simulink model "IEEE_9bus_new_o"  (R2024a)
settings: Solver=ode45  StartTime=0.0  StopTime=60/60  RelTol=1e-3  EnableMultiTasking=on
PreLoadFcn:
  | faultType = "ABCG";
  | faultLineStr = "Line 7-8";
  | faultDistance = 50;
  | L78_Length = 50;
  | L89_Length = 50;
  | L96_Length = 50;
  | L64_Length = 50;
  | L45_Length = 50;
  | L57_Length = 50;
  | 
  | mdl = load('lineIdentificationModel.mat');
  | lineMdl = mdl.treeModel;
  | 
  | mdl = load('typeIdentificationModelV2.mat');
  | typeMdl = mdl.treeModel;
  | 
  | mdl = load('faultLocationModel.mat');
  | locationMdl = mdl.treeModel;
libraries: dspstat3 x36, simulink x24, spsThreePhasePISectionLineLib x12, spsThreePhaseVIMeasurementLib x12, spsLoadFlowBusLib x9, spsThreePhaseFaultLib x6, jailib x3, spsThreePhaseSourceLib x3, spsThreePhaseTransformerTwoWindingsLib x3, statsLibrary x3, spsThreePhaseBreakerLib x3, sps_lib x1
(part 1 of 3)
settings Model: Creator=jp536285  LastModifiedBy=USER
settings SolverCC: AlgebraicLoopSolver=TrustRegion
settings DataIOCC: LimitDataPoints=on  SaveFormat=Array  ReturnWorkspaceOutputs=off
settings OptimizationCC: LifeSpan=inf
settings DebuggingCC: UnderspecifiedInitializationDetection=Classic  MergeDetectMultiDrivingBlocksExec=none  SolverPrmCheckMsg=warning  StateNameClashWarn=warning  SFUnexpectedBacktrackingDiag=warning  SFNoUnconditionalDefaultTransitionDiag=warning  SFExecutionAtInitializationDiag=none  ArithmeticOperatorsInVariantConditions=warning
settings HardwareCC: ProdBitPerPointer=32  ProdBitPerSizeT=32  ProdBitPerPtrDiffT=32  ProdLargestAtomicFloat=None  ProdIntDivRoundTo=Undefined  ProdEndianess=Unspecified  ProdWordSize=32  ProdHWDeviceType=32-bit Generic
settings ModelReferenceCC: EnableParallelModelReferenceBuilds=on  ParallelModelReferenceMATLABWorkerInit=Copy Base Workspace
settings SFSimCC: SimUseLocalCustomCode=off  CustomCodeUndefinedFunction=UseInterfaceOnly
settings RTWCC: RTWUseLocalCustomCode=off  GPUComputeCapability=3.5
settings CodeAppCC: StateflowObjectComments=on
settings GRTTargetCC: TargetLangStandard=C89/C90 (ANSI)
settings ConfigComp: CovMetricSettings=dw  CovSaveCumulativeToWorkspaceVar=on  CovSaveSingleToWorkspaceVar=on  CovExternalEMLEnable=off
settings SimscapeCC: SimscapeNormalizeSystem=off

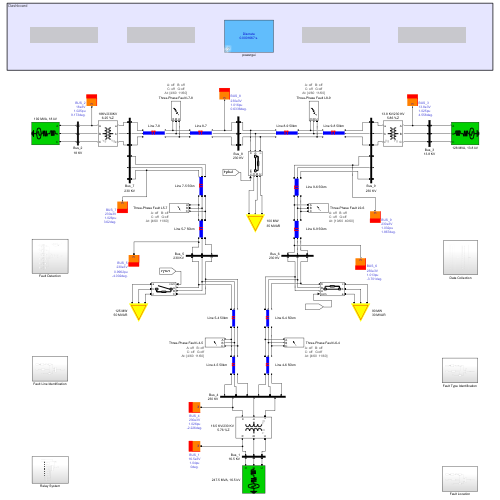
[thumbnail: Simulink's stored preview of the top-level diagram]
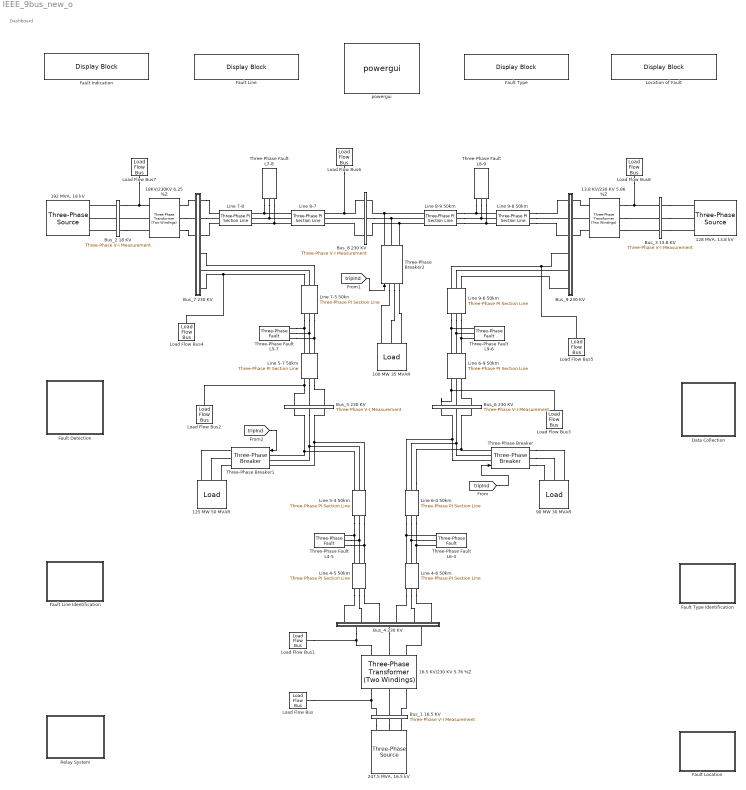
== system IEEE_9bus_new_o ==
  note: Dashboard
  " Line 4-6 50km" : spsThreePhasePISectionLineLib/Three-Phase PI Section Line  LConnTagsString=a|b|c  RConnTagsString=A|B|C  Length=100-L64_Length  Frequency=60  Resistances=[ 0.08993 0.224825]  Inductances="[ 1.29e-3  3.22e-3]"  Capacitances=[7.922e-9 4.74e-9]  mask(Three-Phase PI Section Line){}
      mask Display:
      | % This is a new mask on top of the base mask.
      | % Use "View base mask" link below to see the base mask.
      | patch([0.0 0.0 1 1 0.0 0.0 ],[0.4 0.7 0.7 0.4 0.4 0.7],[0 0 1]);
      | patch([0.4 0.4 0.42 0.42],[0.4 0.75 0.75 0.4],[1 0 0]);
      | patch([0.38 0.38 0.57 0.57],[0.7 0.75 0.75 0.7],[1 0 0]);
      | patch([0.53 0.53 0.55 0.55],[0.4 0.75 0.75 0.4],[1 0 0]);
  " Line 6-4 50km" : spsThreePhasePISectionLineLib/Three-Phase PI Section Line  LConnTagsString=a|b|c  RConnTagsString=A|B|C  Length=L64_Length  Frequency=60  Resistances=[ 0.08993 0.224825]  Inductances="[ 1.29e-3  3.22e-3]"  Capacitances=[7.922e-9 4.74e-9]  mask(Three-Phase PI Section Line){}
      mask Display:
      | % This is a new mask on top of the base mask.
      | % Use "View base mask" link below to see the base mask.
      | patch([0.0 0.0 1 1 0.0 0.0 ],[0.4 0.7 0.7 0.4 0.4 0.7],[0 0 1]);
      | patch([0.4 0.4 0.42 0.42],[0.4 0.75 0.75 0.4],[1 0 0]);
      | patch([0.38 0.38 0.57 0.57],[0.7 0.75 0.75 0.7],[1 0 0]);
      | patch([0.53 0.53 0.55 0.55],[0.4 0.75 0.75 0.4],[1 0 0]);
  " Line 6-9 50km" : spsThreePhasePISectionLineLib/Three-Phase PI Section Line  LConnTagsString=a|b|c  RConnTagsString=A|B|C  Length=100-L96_Length  Frequency=60  Resistances=[ 0.20631 0.5157]  Inductances="[ 2.38e-3  6.09e-3]"  Capacitances=[17.95e-9 10.55e-9]  mask(Three-Phase PI Section Line){}
      mask Display:
      | % This is a new mask on top of the base mask.
      | % Use "View base mask" link below to see the base mask.
      | patch([0.0 0.0 1 1 0.0 0.0 ],[0.4 0.7 0.7 0.4 0.4 0.7],[0 0 1]);
      | patch([0.4 0.4 0.42 0.42],[0.4 0.75 0.75 0.4],[1 0 0]);
      | patch([0.38 0.38 0.57 0.57],[0.7 0.75 0.75 0.7],[1 0 0]);
      | patch([0.53 0.53 0.55 0.55],[0.4 0.75 0.75 0.4],[1 0 0]);
  " Line 9-6 50km" : spsThreePhasePISectionLineLib/Three-Phase PI Section Line  LConnTagsString=a|b|c  RConnTagsString=A|B|C  Length=L96_Length  Frequency=60  Resistances=[ 0.20631 0.5157]  Inductances="[ 2.38e-3  6.09e-3]"  Capacitances=[17.95e-9 10.55e-9]  mask(Three-Phase PI Section Line){}
      mask Display:
      | % This is a new mask on top of the base mask.
      | % Use "View base mask" link below to see the base mask.
      | patch([0.0 0.0 1 1 0.0 0.0 ],[0.4 0.7 0.7 0.4 0.4 0.7],[0 0 1]);
      | patch([0.4 0.4 0.42 0.42],[0.4 0.75 0.75 0.4],[1 0 0]);
      | patch([0.38 0.38 0.57 0.57],[0.7 0.75 0.75 0.7],[1 0 0]);
      | patch([0.53 0.53 0.55 0.55],[0.4 0.75 0.75 0.4],[1 0 0]);
  100 MW 35 MVAR : jailib/Load  SystemSampleTime=-1  VariantActivationTime=update diagram  AllowFlexibleInterface=on  Latency=0  AutoFrameSizeCalculation=off
      link override Three-Phase Parallel RLC Load: NominalVoltage=230000  ActivePower=100e6  InductivePower=35e6
      settings: SourceProductName=Power Library
  125 MW 50 MVAR : jailib/Load  SystemSampleTime=-1  VariantActivationTime=update diagram  AllowFlexibleInterface=on  Latency=0  AutoFrameSizeCalculation=off
      link override Three-Phase Parallel RLC Load: NominalVoltage=230000  ActivePower=125e6  InductivePower=50e6
      settings: SourceProductName=Power Library
  "128 MVA, 13.8 kV" : spsThreePhaseSourceLib/Three-Phase Source  InternalConnection=Yg  VoltagePhases=off  Voltage=13800  PhaseAngle=0  Voltage_phases=[25e3 25e3 25e3]/sqrt(3)  PhaseAngles_phases=[0 -120 +120]  Frequency=60  NonIdealSource=on  SpecifyImpedance=on  Resistance=0.529  Inductance=0.0140  ShortCircuitLevel=128e6  BaseVoltage=13.8e3  XRratio=100000  BusType=PV  Pref=85000000  Qref=0  Prefabc=[10e3, 10e3, 10e3]  Qrefabc=[0, 0, 0]  Qmin=-inf  Qmax=inf
  13.8 KV/230 KV 5.86 %Z : spsThreePhaseTransformerTwoWindingsLib/Three-Phase Transformer (Two Windings)  Winding1Connection=Yg  Winding2Connection=Yg  CoreType=Three single-phase transformers  SetSaturation=off  Hysteresis=off  DataFile='hysteresis'  SetInitialFlux=off  Measurements=None  UNITS=pu  NominalPower=[ 100e6 , 60 ]  Winding1=[ 13.8e3 , 1e-6 , 0 ]  Winding2=[ 230e3 , 1e-6, 0.0586 ]  Rm=500  Lm=500  L0=0.5  Saturation=[ 0,0 ; 0.0024,1.2 ; 1.0,1.52 ]  InitialFluxes=[ 0.8 , -0.8 , 0.7 ]  BreakLoop=off  DiscreteSolver=Trapezoidal iterative  DataType=off  TransfoNumber=1
  "16.5 KV/230 KV 5.76 %Z     " : spsThreePhaseTransformerTwoWindingsLib/Three-Phase Transformer (Two Windings)  Winding1Connection=Yg  Winding2Connection=Yg  CoreType=Three single-phase transformers  SetSaturation=off  Hysteresis=off  DataFile='hysteresis'  SetInitialFlux=off  Measurements=None  UNITS=pu  NominalPower=[ 100e6 , 60 ]  Winding1=[ 16.5e3 , 1e-6, 0 ]  Winding2=[ 230e3 ,1e-6, 0.0576 ]  Rm=500  Lm=500  L0=0.5  Saturation=[ 0,0 ; 0.0024,1.2 ; 1.0,1.52 ]  InitialFluxes=[ 0.8 , -0.8 , 0.7 ]  BreakLoop=off  DiscreteSolver=Trapezoidal iterative  DataType=off  TransfoNumber=1
  18KV/230KV 6.25 %Z : spsThreePhaseTransformerTwoWindingsLib/Three-Phase Transformer (Two Windings)  Winding1Connection=Yg  Winding2Connection=Yg  CoreType=Three single-phase transformers  SetSaturation=off  Hysteresis=off  DataFile='hysteresis'  SetInitialFlux=off  Measurements=None  UNITS=pu  NominalPower=[ 100e6 , 60 ]  Winding1=[ 18e3 , 1e-6 , 0]  Winding2=[ 230e3 , 1e-6, 0.0625 ]  Rm=500  Lm=500  L0=0.5  Saturation=[ 0,0 ; 0.0024,1.2 ; 1.0,1.52 ]  InitialFluxes=[ 0.8 , -0.8 , 0.7 ]  BreakLoop=off  DiscreteSolver=Trapezoidal iterative  DataType=off  TransfoNumber=1
  "192 MVA, 18 kV" : spsThreePhaseSourceLib/Three-Phase Source  InternalConnection=Yg  VoltagePhases=off  Voltage=18000  PhaseAngle=0  Voltage_phases=[25e3 25e3 25e3]/sqrt(3)  PhaseAngles_phases=[0 -120 +120]  Frequency=60  NonIdealSource=on  SpecifyImpedance=on  Resistance=0.529  Inductance=0.0140  ShortCircuitLevel=192e6  BaseVoltage=18e3  XRratio=100000  BusType=PV  Pref=163000000  Qref=0  Prefabc=[10e3, 10e3, 10e3]  Qrefabc=[0, 0, 0]  Qmin=-inf  Qmax=inf
  "247.5 MVA, 16.5 kV" : spsThreePhaseSourceLib/Three-Phase Source  InternalConnection=Yg  VoltagePhases=off  Voltage=16500  PhaseAngle=0  Voltage_phases=[25e3 25e3 25e3]/sqrt(3)  PhaseAngles_phases=[0 -120 +120]  Frequency=60  NonIdealSource=on  SpecifyImpedance=on  Resistance=0.529  Inductance=0.0140  ShortCircuitLevel=247.5e6  BaseVoltage=16.5e3  XRratio=100000  BusType=swing  Pref=0  Qref=0  Prefabc=[10e3, 10e3, 10e3]  Qrefabc=[0, 0, 0]  Qmin=-Inf  Qmax=Inf
  90 MW 30 MVAR : jailib/Load  SystemSampleTime=-1  VariantActivationTime=update diagram  AllowFlexibleInterface=on  Latency=0  AutoFrameSizeCalculation=off
      settings: SourceProductName=Power Library
  Bus_1 16.5 KV : spsThreePhaseVIMeasurementLib/Three-Phase V-I Measurement  VoltageMeasurement=phase-to-ground  SetLabelV=on  LabelV=Vabc_1  Vpu=on  VpuLL=off  CurrentMeasurement=yes  SetLabelI=on  LabelI=Iabc_1  Ipu=on  Pbase=100e6  Vbase=16.5e3  OutputType=Complex  PhasorSimulation=off  PSBequivalent=0
  Bus_2 18 KV : spsThreePhaseVIMeasurementLib/Three-Phase V-I Measurement  VoltageMeasurement=phase-to-ground  SetLabelV=on  LabelV=Vabc_2  Vpu=on  VpuLL=off  CurrentMeasurement=yes  SetLabelI=on  LabelI=Iabc_2  Ipu=on  Pbase=100e6  Vbase=18e3  OutputType=Complex  PhasorSimulation=off  PSBequivalent=0
  Bus_3 13.8 KV : spsThreePhaseVIMeasurementLib/Three-Phase V-I Measurement  VoltageMeasurement=phase-to-ground  SetLabelV=on  LabelV=Vabc_3  Vpu=on  VpuLL=off  CurrentMeasurement=yes  SetLabelI=on  LabelI=Iabc_3  Ipu=on  Pbase=100e6  Vbase=13.8e3  OutputType=Complex  PhasorSimulation=off  PSBequivalent=0
  Bus_4 230 KV : Subsystem
  Bus_5 230 KV : spsThreePhaseVIMeasurementLib/Three-Phase V-I Measurement  VoltageMeasurement=phase-to-ground  SetLabelV=on  LabelV=Vabc_5  Vpu=on  VpuLL=off  CurrentMeasurement=yes  SetLabelI=on  LabelI=Iabc_5  Ipu=on  Pbase=100e6  Vbase=230e3  OutputType=Complex  PhasorSimulation=off  PSBequivalent=0
  Bus_6 230 KV : spsThreePhaseVIMeasurementLib/Three-Phase V-I Measurement  VoltageMeasurement=phase-to-ground  SetLabelV=on  LabelV=Vabc_6  Vpu=on  VpuLL=off  CurrentMeasurement=yes  SetLabelI=on  LabelI=Iabc_6  Ipu=on  Pbase=100e6  Vbase=230e3  OutputType=Complex  PhasorSimulation=off  PSBequivalent=0
  Bus_7 230 KV : Subsystem
  Bus_8 230 KV : spsThreePhaseVIMeasurementLib/Three-Phase V-I Measurement  VoltageMeasurement=phase-to-ground  SetLabelV=on  LabelV=Vabc_8  Vpu=on  VpuLL=off  CurrentMeasurement=yes  SetLabelI=on  LabelI=Iabc_8  Ipu=on  Pbase=100e6  Vbase=230e3  OutputType=Complex  PhasorSimulation=off  PSBequivalent=0
  Bus_9 230 KV : Subsystem
  Data Collection : Subsystem
  Fault Detection : Subsystem
  Fault Indication : DisplayBlock  LabelPosition=Hide  Transparency=1  Layout=Fill available space
  Fault Line : DisplayBlock  LabelPosition=Hide  Transparency=1
  Fault Line Identification : Subsystem
  Fault Location : Subsystem
  Fault Type : DisplayBlock  LabelPosition=Hide  Transparency=1
  Fault Type Identification : Subsystem
  "Line 4-5 50km " : spsThreePhasePISectionLineLib/Three-Phase PI Section Line  LConnTagsString=a|b|c  RConnTagsString=A|B|C  Length=L45_Length  Frequency=60  Resistances=[ 0.0529 0.13225]  Inductances="[ 1.192e-3  2.38e-3]"  Capacitances=[8.82e-9 5.188e-9]  mask(Three-Phase PI Section Line){}
      mask Display:
      | % This is a new mask on top of the base mask.
      | % Use "View base mask" link below to see the base mask.
      | patch([0.0 0.0 1 1 0.0 0.0 ],[0.4 0.7 0.7 0.4 0.4 0.7],[0 0 1]);
      | patch([0.4 0.4 0.42 0.42],[0.4 0.75 0.75 0.4],[1 0 0]);
      | patch([0.38 0.38 0.57 0.57],[0.7 0.75 0.75 0.7],[1 0 0]);
      | patch([0.53 0.53 0.55 0.55],[0.4 0.75 0.75 0.4],[1 0 0]);
  Line 5-4 50km : spsThreePhasePISectionLineLib/Three-Phase PI Section Line  LConnTagsString=a|b|c  RConnTagsString=A|B|C  Length=100-L45_Length  Frequency=60  Resistances=[ 0.0529 0.13225]  Inductances="[ 1.192e-3  2.38e-3]"  Capacitances=[8.82e-9 5.188e-9]  mask(Three-Phase PI Section Line){}
      mask Display:
      | % This is a new mask on top of the base mask.
      | % Use "View base mask" link below to see the base mask.
      | patch([0.0 0.0 1 1 0.0 0.0 ],[0.4 0.7 0.7 0.4 0.4 0.7],[0 0 1]);
      | patch([0.4 0.4 0.42 0.42],[0.4 0.75 0.75 0.4],[1 0 0]);
      | patch([0.38 0.38 0.57 0.57],[0.7 0.75 0.75 0.7],[1 0 0]);
      | patch([0.53 0.53 0.55 0.55],[0.4 0.75 0.75 0.4],[1 0 0]);
  Line 5-7 50km : spsThreePhasePISectionLineLib/Three-Phase PI Section Line  LConnTagsString=a|b|c  RConnTagsString=A|B|C  Length=L57_Length  Frequency=60  Resistances=[ 0.16928 0.4232]  Inductances="[ 2.259e-3  5.64e-3]"  Capacitances=[15.34e-9 9.025e-9]  mask(Three-Phase PI Section Line){}
      mask Display:
      | % This is a new mask on top of the base mask.
      | % Use "View base mask" link below to see the base mask.
      | patch([0.0 0.0 1 1 0.0 0.0 ],[0.4 0.7 0.7 0.4 0.4 0.7],[0 0 1]);
      | patch([0.4 0.4 0.42 0.42],[0.4 0.75 0.75 0.4],[1 0 0]);
      | patch([0.38 0.38 0.57 0.57],[0.7 0.75 0.75 0.7],[1 0 0]);
      | patch([0.53 0.53 0.55 0.55],[0.4 0.75 0.75 0.4],[1 0 0]);
  Line 7-5 50kn : spsThreePhasePISectionLineLib/Three-Phase PI Section Line  LConnTagsString=a|b|c  RConnTagsString=A|B|C  Length=100-L57_Length  Frequency=60  Resistances=[ 0.16928 0.4232]  Inductances="[ 2.259e-3  5.64e-3]"  Capacitances=[15.34e-9 9.025e-9]  mask(Three-Phase PI Section Line){}
      mask Display:
      | % This is a new mask on top of the base mask.
      | % Use "View base mask" link below to see the base mask.
      | patch([0.0 0.0 1 1 0.0 0.0 ],[0.4 0.7 0.7 0.4 0.4 0.7],[0 0 1]);
      | patch([0.4 0.4 0.42 0.42],[0.4 0.75 0.75 0.4],[1 0 0]);
      | patch([0.38 0.38 0.57 0.57],[0.7 0.75 0.75 0.7],[1 0 0]);
      | patch([0.53 0.53 0.55 0.55],[0.4 0.75 0.75 0.4],[1 0 0]);
  Line 7-8 : spsThreePhasePISectionLineLib/Three-Phase PI Section Line  LConnTagsString=a|b|c  RConnTagsString=A|B|C  Length=L78_Length  Frequency=60  Resistances=[0.044965 0.11241]  Inductances="[ 1.01e-3  2.02e-3]"  Capacitances=[7.471e-9 4.394e-9]  mask(Three-Phase PI Section Line){}
      mask Display:
      | % This is a new mask on top of the base mask.
      | % Use "View base mask" link below to see the base mask.
      | patch([0.0 0.0 1 1 0.0 0.0 ],[0.4 0.7 0.7 0.4 0.4 0.7],[0 0 1]);
      | patch([0.4 0.4 0.42 0.42],[0.4 0.75 0.75 0.4],[1 0 0]);
      | patch([0.38 0.38 0.57 0.57],[0.7 0.75 0.75 0.7],[1 0 0]);
      | patch([0.53 0.53 0.55 0.55],[0.4 0.75 0.75 0.4],[1 0 0]);
  Line 8-7 : spsThreePhasePISectionLineLib/Three-Phase PI Section Line  LConnTagsString=a|b|c  RConnTagsString=A|B|C  Length=100 - L78_Length  Frequency=60  Resistances=[0.044965 0.11241]  Inductances="[ 1.01e-3  2.02e-3]"  Capacitances=[7.471e-9 4.394e-9]  mask(Three-Phase PI Section Line){}
      mask Display:
      | % This is a new mask on top of the base mask.
      | % Use "View base mask" link below to see the base mask.
      | patch([0.0 0.0 1 1 0.0 0.0 ],[0.4 0.7 0.7 0.4 0.4 0.7],[0 0 1]);
      | patch([0.4 0.4 0.42 0.42],[0.4 0.75 0.75 0.4],[1 0 0]);
      | patch([0.38 0.38 0.57 0.57],[0.7 0.75 0.75 0.7],[1 0 0]);
      | patch([0.53 0.53 0.55 0.55],[0.4 0.75 0.75 0.4],[1 0 0]);
  Line 8-9 50km : spsThreePhasePISectionLineLib/Three-Phase PI Section Line  LConnTagsString=a|b|c  RConnTagsString=A|B|C  Length=L89_Length  Frequency=60  Resistances=[ 0.062951 0.15737]  Inductances="[ 1.414e-3  3.53e-3]"  Capacitances=[10.47e-9 6.15e-9]  mask(Three-Phase PI Section Line){}
      mask Display:
      | % This is a new mask on top of the base mask.
      | % Use "View base mask" link below to see the base mask.
      | patch([0.0 0.0 1 1 0.0 0.0 ],[0.4 0.7 0.7 0.4 0.4 0.7],[0 0 1]);
      | patch([0.4 0.4 0.42 0.42],[0.4 0.75 0.75 0.4],[1 0 0]);
      | patch([0.38 0.38 0.57 0.57],[0.7 0.75 0.75 0.7],[1 0 0]);
      | patch([0.53 0.53 0.55 0.55],[0.4 0.75 0.75 0.4],[1 0 0]);
  Line 9-8 50km : spsThreePhasePISectionLineLib/Three-Phase PI Section Line  LConnTagsString=a|b|c  RConnTagsString=A|B|C  Length=100-L89_Length  Frequency=60  Resistances=[ 0.062951 0.15737]  Inductances="[ 1.414e-3  3.53e-3]"  Capacitances=[10.47e-9 6.15e-9]  mask(Three-Phase PI Section Line){}
      mask Display:
      | % This is a new mask on top of the base mask.
      | % Use "View base mask" link below to see the base mask.
      | patch([0.0 0.0 1 1 0.0 0.0 ],[0.4 0.7 0.7 0.4 0.4 0.7],[0 0 1]);
      | patch([0.4 0.4 0.42 0.42],[0.4 0.75 0.75 0.4],[1 0 0]);
      | patch([0.38 0.38 0.57 0.57],[0.7 0.75 0.75 0.7],[1 0 0]);
      | patch([0.53 0.53 0.55 0.55],[0.4 0.75 0.75 0.4],[1 0 0]);
  Load Flow Bus : spsLoadFlowBusLib/Load Flow Bus  LConnTagsString=a  Phases=single  Connectors=on one side  ID=BUS_1  Vbase=16.5e3  Vref=1.04  Vangle=0  VLF=1.04  VLFb=1  VLFc=1  angleLF=0  angleLFb=0  angleLFc=0
      settings: AttributesFormatString=%<ID>\n%<Vbase>V\n%<VLF>pu\n%<angleLF>deg.
  Load Flow Bus1 : spsLoadFlowBusLib/Load Flow Bus  LConnTagsString=a  Phases=single  Connectors=on one side  ID=BUS_4  Vbase=230e3  Vref=1  Vangle=0  VLF=1.026  VLFb=1  VLFc=1  angleLF=-2.226  angleLFb=0  angleLFc=0
      settings: AttributesFormatString=%<ID>\n%<Vbase>V\n%<VLF>pu\n%<angleLF>deg.
  Load Flow Bus2 : spsLoadFlowBusLib/Load Flow Bus  LConnTagsString=a  Phases=single  Connectors=on one side  ID=BUS_5  Vbase=230e3  Vref=1  Vangle=0  VLF=0.9962  VLFb=1  VLFc=1  angleLF=-4.002  angleLFb=0  angleLFc=0
      settings: AttributesFormatString=%<ID>\n%<Vbase>V\n%<VLF>pu\n%<angleLF>deg.
  Load Flow Bus3 : spsLoadFlowBusLib/Load Flow Bus  LConnTagsString=a  Phases=single  Connectors=on one side  ID=BUS_6  Vbase=230e3  Vref=1  Vangle=0  VLF=1.013  VLFb=1  VLFc=1  angleLF=-3.701  angleLFb=0  angleLFc=0
      settings: AttributesFormatString=%<ID>\n%<Vbase>V\n%<VLF>pu\n%<angleLF>deg.
  Load Flow Bus4 : spsLoadFlowBusLib/Load Flow Bus  LConnTagsString=a  Phases=single  Connectors=on one side  ID=BUS_7  Vbase=230e3  Vref=1  Vangle=0  VLF=1.026  VLFb=1  VLFc=1  angleLF=3.62  angleLFb=0  angleLFc=0
      settings: AttributesFormatString=%<ID>\n%<Vbase>V\n%<VLF>pu\n%<angleLF>deg.
  Load Flow Bus5 : spsLoadFlowBusLib/Load Flow Bus  LConnTagsString=a  Phases=single  Connectors=on one side  ID=BUS_9  Vbase=230e3  Vref=1  Vangle=0  VLF=1.032  VLFb=1  VLFc=1  angleLF=1.867  angleLFb=0  angleLFc=0
      settings: AttributesFormatString=%<ID>\n%<Vbase>V\n%<VLF>pu\n%<angleLF>deg.
  Load Flow Bus6 : spsLoadFlowBusLib/Load Flow Bus  LConnTagsString=a  Phases=single  Connectors=on one side  ID=BUS_8  Vbase=230e3  Vref=1  Vangle=0  VLF=1.016  VLFb=1  VLFc=1  angleLF=0.6336  angleLFb=0  angleLFc=0
      settings: AttributesFormatString=%<ID>\n%<Vbase>V\n%<VLF>pu\n%<angleLF>deg.
  Load Flow Bus7 : spsLoadFlowBusLib/Load Flow Bus  LConnTagsString=a  Phases=single  Connectors=on one side  ID=BUS_2  Vbase=18e3  Vref=1.025  Vangle=0  VLF=1.025  VLFb=1  VLFc=1  angleLF=9.173  angleLFb=0  angleLFc=0
      settings: AttributesFormatString=%<ID>\n%<Vbase>V\n%<VLF>pu\n%<angleLF>deg.
  Load Flow Bus8 : spsLoadFlowBusLib/Load Flow Bus  LConnTagsString=a  Phases=single  Connectors=on one side  ID=BUS_3  Vbase=13.8e3  Vref=1.025  Vangle=0  VLF=1.025  VLFb=1  VLFc=1  angleLF=4.558  angleLFb=0  angleLFc=0
      settings: AttributesFormatString=%<ID>\n%<Vbase>V\n%<VLF>pu\n%<angleLF>deg.
  Location of Fault : DisplayBlock  LabelPosition=Hide  Transparency=1
  Relay System : Subsystem
  Three-Phase Breaker : spsThreePhaseBreakerLib/Three-Phase Breaker  InitialState=closed  SwitchA=off  SwitchB=off  SwitchC=off  SwitchTimes="[1/60  5/60]"  External=on  BreakerResistance=0.01  SnubberResistance=1e6  SnubberCapacitance=inf  Measurements=None
  Three-Phase Breaker1 : spsThreePhaseBreakerLib/Three-Phase Breaker  InitialState=open  SwitchA=off  SwitchB=off  SwitchC=off  SwitchTimes="[0/60  14/60]"  External=on  BreakerResistance=0.01  SnubberResistance=1e6  SnubberCapacitance=inf  Measurements=None
  Three-Phase Breaker2 : spsThreePhaseBreakerLib/Three-Phase Breaker  InitialState=closed  SwitchA=off  SwitchB=off  SwitchC=off  SwitchTimes="[1/60  5/60]"  External=on  BreakerResistance=0.01  SnubberResistance=1e6  SnubberCapacitance=inf  Measurements=None
  Three-Phase Fault L4-5 : spsThreePhaseFaultLib/Three-Phase Fault  InitialStates=0  FaultA=off  FaultB=off  FaultC=off  GroundFault=off  SwitchTimes="[4/60  11/60]"  External=off  SwitchStatus=NaN  FaultResistance=0.001  GroundResistance=0.01  SnubberResistance=1e6  SnubberCapacitance=inf  Measurements=None
      settings: AttributesFormatString=|
      | A: %<FaultA>   B: %<FaultB>
      | C: %<FaultC>   G:%<GroundFault>
      | At: %<SwitchTimes>
  Three-Phase Fault L5-7 : spsThreePhaseFaultLib/Three-Phase Fault  InitialStates=0  FaultA=off  FaultB=off  FaultC=off  GroundFault=off  SwitchTimes="[4/60  11/60]"  External=off  SwitchStatus=NaN  FaultResistance=0.001  GroundResistance=0.01  SnubberResistance=1e6  SnubberCapacitance=inf  Measurements=None
      settings: AttributesFormatString=|
      | A: %<FaultA>   B: %<FaultB>
      | C: %<FaultC>   G:%<GroundFault>
      | At: %<SwitchTimes>
  Three-Phase Fault L6-4 : spsThreePhaseFaultLib/Three-Phase Fault  InitialStates=0  FaultA=off  FaultB=off  FaultC=off  GroundFault=off  SwitchTimes="[4/60  11/60]"  External=off  SwitchStatus=NaN  FaultResistance=0.001  GroundResistance=0.01  SnubberResistance=1e6  SnubberCapacitance=inf  Measurements=None
      settings: AttributesFormatString=|
      | A: %<FaultA>   B: %<FaultB>
      | C: %<FaultC>   G:%<GroundFault>
      | At: %<SwitchTimes>
  Three-Phase Fault L7-8 : spsThreePhaseFaultLib/Three-Phase Fault  InitialStates=0  FaultA=off  FaultB=off  FaultC=off  GroundFault=off  SwitchTimes="[4/60  11/60]"  External=off  SwitchStatus=NaN  FaultResistance=0.001  GroundResistance=0.01  SnubberResistance=1e6  SnubberCapacitance=inf  Measurements=None
      settings: AttributesFormatString=|
      | A: %<FaultA>   B: %<FaultB>
      | C: %<FaultC>   G:%<GroundFault>
      | At: %<SwitchTimes>
  Three-Phase Fault L8-9 : spsThreePhaseFaultLib/Three-Phase Fault  InitialStates=0  FaultA=off  FaultB=off  FaultC=off  GroundFault=off  SwitchTimes="[4/60  11/60]"  External=off  SwitchStatus=NaN  FaultResistance=0.001  GroundResistance=0.01  SnubberResistance=1e6  SnubberCapacitance=inf  Measurements=None
      settings: AttributesFormatString=|
      | A: %<FaultA>   B: %<FaultB>
      | C: %<FaultC>   G:%<GroundFault>
      | At: %<SwitchTimes>
  Three-Phase Fault L9-6 : spsThreePhaseFaultLib/Three-Phase Fault  InitialStates=0  FaultA=off  FaultB=off  FaultC=off  GroundFault=off  SwitchTimes="[10/60  40/60]"  External=off  SwitchStatus=NaN  FaultResistance=0.001  GroundResistance=0.01  SnubberResistance=1e6  SnubberCapacitance=inf  Measurements=None
      settings: AttributesFormatString=|
      | A: %<FaultA>   B: %<FaultB>
      | C: %<FaultC>   G:%<GroundFault>
      | At: %<SwitchTimes>
  powergui : sps_lib/powergui  Priority=1  SimulationMode=Discrete  SampleTime=(1/6)*10^(-3)  frequency=60  Iterations=50  frequencyindice=60  Pbase=10e7  ErrMax=1e-05  UnitsV=kV  UnitsW=MW  buscounter=0  FunctionMessages=off  echomessages=off  EnableUseOfTLC=off  CurrentSourceSwitches=off  DisableSnubberDevices=off  DisableRonSwitches=off  DisableVfSwitches=off  DisplayEquations=off  AutomaticDiscreteSolvers=off  SolverType=Tustin  Interpol=off  ExternalGateDelay=off  methode=off  Ts=0  x0status=blocks  SPID=off  SwTol=0  HookPort=off  NonlinearTolerance=1e-4  nMaxIteration=100  ContinueOnMaxIteration=off  RestoreLinks=warning  ResistiveCurrentMeasurement=off  Frange=[0:2:500]  Ylog=off  Xlog=on  ShowGrid=off  save=off  variable=ZData  structure=0  ZoomFFT=off  StartTime=0.0  cycles=1  DisplayStyle=1  fundamental=60  FreqAxis=off  MaxFrequency=1000  frequencyindicesteady=1  RmsSteady=1  display=off
  wires:
  [tripInd] -> Three-Phase Breaker/1
  [tripInd] -> Three-Phase Breaker2/1
  [tripInd] -> Three-Phase Breaker1/1
  connections:
  Bus_2 18 KV/LConn2 -- "192 MVA, 18 kV"/RConn2
  18KV/230KV 6.25 %Z/LConn2 -- Bus_2 18 KV/RConn2
  18KV/230KV 6.25 %Z/RConn2 -- Bus_7 230 KV/LConn2
  Bus_2 18 KV/RConn1 -- Load Flow Bus7/LConn1 -- 18KV/230KV 6.25 %Z/LConn1
  Bus_2 18 KV/RConn3 -- 18KV/230KV 6.25 %Z/LConn3
  Bus_7 230 KV/LConn1 -- 18KV/230KV 6.25 %Z/RConn1
  18KV/230KV 6.25 %Z/RConn3 -- Bus_7 230 KV/LConn3
  Load Flow Bus8/LConn1 -- Bus_3 13.8 KV/LConn1 -- 13.8 KV/230 KV 5.86 %Z/LConn1
  13.8 KV/230 KV 5.86 %Z/LConn2 -- Bus_3 13.8 KV/LConn2
  13.8 KV/230 KV 5.86 %Z/LConn3 -- Bus_3 13.8 KV/LConn3
  Bus_1 16.5 KV/RConn1 -- "247.5 MVA, 16.5 kV"/RConn1
  Bus_1 16.5 KV/RConn2 -- "247.5 MVA, 16.5 kV"/RConn2
  Bus_1 16.5 KV/RConn3 -- "247.5 MVA, 16.5 kV"/RConn3
  Bus_1 16.5 KV/LConn1 -- Load Flow Bus/LConn1 -- "16.5 KV/230 KV 5.76 %Z     "/LConn1
  Bus_1 16.5 KV/LConn3 -- "16.5 KV/230 KV 5.76 %Z     "/LConn3
  Bus_1 16.5 KV/LConn2 -- "16.5 KV/230 KV 5.76 %Z     "/LConn2
  13.8 KV/230 KV 5.86 %Z/RConn1 -- Bus_9 230 KV/RConn1
  13.8 KV/230 KV 5.86 %Z/RConn2 -- Bus_9 230 KV/RConn2
  13.8 KV/230 KV 5.86 %Z/RConn3 -- Bus_9 230 KV/RConn3
  Bus_4 230 KV/LConn1 -- "16.5 KV/230 KV 5.76 %Z     "/RConn1 -- Load Flow Bus1/LConn1
  Bus_4 230 KV/LConn2 -- "16.5 KV/230 KV 5.76 %Z     "/RConn2
  Line 8-9 50km/LConn1 -- Three-Phase Breaker2/RConn1 -- Bus_8 230 KV/LConn1
  Bus_8 230 KV/LConn2 -- Line 8-9 50km/LConn2 -- Three-Phase Breaker2/RConn2
  Line 8-9 50km/LConn3 -- Bus_8 230 KV/LConn3 -- Three-Phase Breaker2/RConn3
  "16.5 KV/230 KV 5.76 %Z     "/RConn3 -- Bus_4 230 KV/LConn3
  Bus_6 230 KV/RConn1 -- Three-Phase Breaker/LConn1 -- " Line 6-4 50km"/LConn1
  Bus_6 230 KV/RConn2 -- Three-Phase Breaker/LConn2 -- " Line 6-4 50km"/LConn2
  " Line 6-4 50km"/LConn3 -- Bus_6 230 KV/RConn3 -- Three-Phase Breaker/LConn3
  Line 9-8 50km/RConn2 -- Bus_9 230 KV/LConn2
  Line 9-8 50km/RConn1 -- Bus_9 230 KV/LConn1
  Line 9-8 50km/RConn3 -- Bus_9 230 KV/LConn3
  Line 5-7 50km/RConn1 -- Load Flow Bus2/LConn1 -- Bus_5 230 KV/LConn1
  Line 5-7 50km/RConn2 -- Bus_5 230 KV/LConn2
  Line 5-7 50km/RConn3 -- Bus_5 230 KV/LConn3
  Load Flow Bus4/LConn1 -- Line 7-5 50kn/LConn1 -- Bus_7 230 KV/RConn6
  Line 7-5 50kn/LConn2 -- Bus_7 230 KV/RConn5
  Bus_7 230 KV/RConn4 -- Line 7-5 50kn/LConn3
  Bus_9 230 KV/LConn5 -- " Line 9-6 50km"/RConn2
  Bus_6 230 KV/LConn1 -- Load Flow Bus3/LConn1 -- " Line 6-9 50km"/LConn1
  Bus_6 230 KV/LConn2 -- " Line 6-9 50km"/LConn2
  Bus_6 230 KV/LConn3 -- " Line 6-9 50km"/LConn3
  Load Flow Bus5/LConn1 -- Bus_9 230 KV/LConn4 -- " Line 9-6 50km"/RConn1
  "Line 4-5 50km "/RConn2 -- Bus_4 230 KV/RConn2
  "Line 4-5 50km "/RConn1 -- Bus_4 230 KV/RConn1
  "Line 4-5 50km "/RConn3 -- Bus_4 230 KV/RConn3
  " Line 4-6 50km"/RConn2 -- Bus_4 230 KV/RConn5
  " Line 4-6 50km"/RConn1 -- Bus_4 230 KV/RConn4
  " Line 4-6 50km"/RConn3 -- Bus_4 230 KV/RConn6
  Bus_3 13.8 KV/RConn1 -- "128 MVA, 13.8 kV"/RConn1
  Bus_3 13.8 KV/RConn2 -- "128 MVA, 13.8 kV"/RConn2
  Bus_3 13.8 KV/RConn3 -- "128 MVA, 13.8 kV"/RConn3
  Bus_2 18 KV/LConn3 -- "192 MVA, 18 kV"/RConn3
  Bus_2 18 KV/LConn1 -- "192 MVA, 18 kV"/RConn1
  Bus_8 230 KV/RConn2 -- Line 8-7/RConn2
  Bus_8 230 KV/RConn1 -- Load Flow Bus6/LConn1 -- Line 8-7/RConn1
  Bus_8 230 KV/RConn3 -- Line 8-7/RConn3
  Bus_7 230 KV/RConn1 -- Line 7-8/LConn1
  Bus_7 230 KV/RConn2 -- Line 7-8/LConn2
  Bus_7 230 KV/RConn3 -- Line 7-8/LConn3
  Line 8-7/LConn2 -- Three-Phase Fault L7-8/LConn2 -- Line 7-8/RConn2
  Line 8-7/LConn1 -- Three-Phase Fault L7-8/LConn1 -- Line 7-8/RConn1
  Line 8-7/LConn3 -- Three-Phase Fault L7-8/LConn3 -- Line 7-8/RConn3
  Three-Phase Fault L8-9/LConn2 -- Line 8-9 50km/RConn2 -- Line 9-8 50km/LConn2
  Three-Phase Fault L8-9/LConn1 -- Line 8-9 50km/RConn1 -- Line 9-8 50km/LConn1
  Three-Phase Fault L8-9/LConn3 -- Line 8-9 50km/RConn3 -- Line 9-8 50km/LConn3
  Line 7-5 50kn/RConn3 -- Line 5-7 50km/LConn3 -- Three-Phase Fault L5-7/LConn3
  Line 7-5 50kn/RConn2 -- Three-Phase Fault L5-7/LConn2 -- Line 5-7 50km/LConn2
  Line 7-5 50kn/RConn1 -- Three-Phase Fault L5-7/LConn1 -- Line 5-7 50km/LConn1
  Bus_9 230 KV/LConn6 -- " Line 9-6 50km"/RConn3
  " Line 9-6 50km"/LConn3 -- Three-Phase Fault L9-6/LConn3 -- " Line 6-9 50km"/RConn3
  " Line 9-6 50km"/LConn2 -- Three-Phase Fault L9-6/LConn2 -- " Line 6-9 50km"/RConn2
  " Line 9-6 50km"/LConn1 -- Three-Phase Fault L9-6/LConn1 -- " Line 6-9 50km"/RConn1
  Line 5-4 50km/RConn2 -- Three-Phase Fault L4-5/LConn2 -- "Line 4-5 50km "/LConn2
  Line 5-4 50km/RConn3 -- Three-Phase Fault L4-5/LConn3 -- "Line 4-5 50km "/LConn3
  Line 5-4 50km/RConn1 -- Three-Phase Fault L4-5/LConn1 -- "Line 4-5 50km "/LConn1
  " Line 6-4 50km"/RConn3 -- Three-Phase Fault L6-4/LConn3 -- " Line 4-6 50km"/LConn3
  " Line 6-4 50km"/RConn2 -- Three-Phase Fault L6-4/LConn2 -- " Line 4-6 50km"/LConn2
  " Line 6-4 50km"/RConn1 -- Three-Phase Fault L6-4/LConn1 -- " Line 4-6 50km"/LConn1
  Bus_5 230 KV/RConn1 -- Line 5-4 50km/LConn1 -- Three-Phase Breaker1/LConn1
  Bus_5 230 KV/RConn2 -- Three-Phase Breaker1/LConn2 -- Line 5-4 50km/LConn2
  Bus_5 230 KV/RConn3 -- Three-Phase Breaker1/LConn3 -- Line 5-4 50km/LConn3
  Three-Phase Breaker/RConn1 -- 90 MW 30 MVAR/LConn1
  Three-Phase Breaker/RConn2 -- 90 MW 30 MVAR/LConn2
  Three-Phase Breaker/RConn3 -- 90 MW 30 MVAR/LConn3
  Three-Phase Breaker1/RConn1 -- 125 MW 50 MVAR/LConn1
  Three-Phase Breaker1/RConn2 -- 125 MW 50 MVAR/LConn2
  Three-Phase Breaker1/RConn3 -- 125 MW 50 MVAR/LConn3
  Three-Phase Breaker2/LConn3 -- 100 MW 35 MVAR/LConn3
  Three-Phase Breaker2/LConn2 -- 100 MW 35 MVAR/LConn2
  Three-Phase Breaker2/LConn1 -- 100 MW 35 MVAR/LConn1

== system IEEE_9bus_new_o/Bus_4 230 KV ==
  Three-Phase V-I Measurement1 : spsThreePhaseVIMeasurementLib/Three-Phase V-I Measurement  VoltageMeasurement=phase-to-ground  SetLabelV=on  LabelV=Vabc_45  Vpu=on  VpuLL=off  CurrentMeasurement=yes  SetLabelI=on  LabelI=Iabc_45  Ipu=on  Pbase=100e6  Vbase=230e3  OutputType=Complex  PhasorSimulation=off  PSBequivalent=0
  Three-Phase V-I Measurement3 : spsThreePhaseVIMeasurementLib/Three-Phase V-I Measurement  VoltageMeasurement=phase-to-ground  SetLabelV=on  LabelV=Vabc_46  Vpu=on  VpuLL=off  CurrentMeasurement=yes  SetLabelI=on  LabelI=Iabc_46  Ipu=on  Pbase=100e6  Vbase=230e3  OutputType=Complex  PhasorSimulation=off  PSBequivalent=0
  Conn7 : PMIOPort  Side=Left
  Conn8 : PMIOPort  Port=2  Side=Left
  Conn9 : PMIOPort  Port=3  Side=Left
  Conn1 : PMIOPort  Port=4  Side=Right
  Conn2 : PMIOPort  Port=5  Side=Right
  Conn3 : PMIOPort  Port=6  Side=Right
  Conn4 : PMIOPort  Port=7  Side=Right
  Conn5 : PMIOPort  Port=8  Side=Right
  Conn6 : PMIOPort  Port=9  Side=Right
  connections:
  Three-Phase V-I Measurement3/LConn3 -- Conn9/RConn1 -- Three-Phase V-I Measurement1/LConn3
  Three-Phase V-I Measurement3/LConn2 -- Conn8/RConn1 -- Three-Phase V-I Measurement1/LConn2
  Three-Phase V-I Measurement3/LConn1 -- Conn7/RConn1 -- Three-Phase V-I Measurement1/LConn1
  Three-Phase V-I Measurement3/RConn3 -- Conn6/RConn1
  Three-Phase V-I Measurement1/RConn3 -- Conn3/RConn1
  Three-Phase V-I Measurement1/RConn1 -- Conn1/RConn1
  Three-Phase V-I Measurement1/RConn2 -- Conn2/RConn1
  Three-Phase V-I Measurement3/RConn1 -- Conn4/RConn1
  Three-Phase V-I Measurement3/RConn2 -- Conn5/RConn1

== system IEEE_9bus_new_o/Bus_7 230 KV ==
  Three-Phase V-I Measurement1 : spsThreePhaseVIMeasurementLib/Three-Phase V-I Measurement  VoltageMeasurement=phase-to-ground  SetLabelV=on  LabelV=Vabc_7  Vpu=on  VpuLL=off  CurrentMeasurement=yes  SetLabelI=on  LabelI=Iabc_7  Ipu=on  Pbase=100e6  Vbase=230e3  OutputType=Complex  PhasorSimulation=off  PSBequivalent=0
  Three-Phase V-I Measurement3 : spsThreePhaseVIMeasurementLib/Three-Phase V-I Measurement  VoltageMeasurement=phase-to-ground  SetLabelV=on  LabelV=Vab  Vpu=on  VpuLL=off  CurrentMeasurement=yes  SetLabelI=on  LabelI=Iab  Ipu=on  Pbase=100e6  Vbase=230e3  OutputType=Complex  PhasorSimulation=off  PSBequivalent=0
  Conn7 : PMIOPort  Side=Left
  Conn8 : PMIOPort  Port=2  Side=Left
  Conn9 : PMIOPort  Port=3  Side=Left
  Conn1 : PMIOPort  Port=4  Side=Right
  Conn2 : PMIOPort  Port=5  Side=Right
  Conn3 : PMIOPort  Port=6  Side=Right
  Conn4 : PMIOPort  Port=7  Side=Right
  Conn5 : PMIOPort  Port=8  Side=Right
  Conn6 : PMIOPort  Port=9  Side=Right
  Conn10 : PMIOPort  Port=10  Side=Left
  Conn11 : PMIOPort  Port=11  Side=Left
  Conn12 : PMIOPort  Port=12  Side=Left
  connections:
  Three-Phase V-I Measurement3/RConn2 -- Conn5/RConn1
  Three-Phase V-I Measurement3/RConn1 -- Conn4/RConn1
  Three-Phase V-I Measurement1/RConn2 -- Conn2/RConn1
  Three-Phase V-I Measurement1/RConn1 -- Conn1/RConn1
  Three-Phase V-I Measurement1/RConn3 -- Conn3/RConn1
  Three-Phase V-I Measurement3/RConn3 -- Conn6/RConn1
  Conn7/RConn1 -- Three-Phase V-I Measurement3/LConn3 -- Conn12/RConn1 -- Three-Phase V-I Measurement1/LConn1
  Conn8/RConn1 -- Three-Phase V-I Measurement3/LConn2 -- Conn11/RConn1 -- Three-Phase V-I Measurement1/LConn2
  Conn9/RConn1 -- Conn10/RConn1 -- Three-Phase V-I Measurement3/LConn1 -- Three-Phase V-I Measurement1/LConn3

== system IEEE_9bus_new_o/Bus_9 230 KV ==
  Three-Phase V-I Measurement1 : spsThreePhaseVIMeasurementLib/Three-Phase V-I Measurement  VoltageMeasurement=phase-to-ground  SetLabelV=on  LabelV=Vabc_9  Vpu=on  VpuLL=off  CurrentMeasurement=yes  SetLabelI=on  LabelI=Iabc_9  Ipu=on  Pbase=100e6  Vbase=230e3  OutputType=Complex  PhasorSimulation=off  PSBequivalent=0
  Three-Phase V-I Measurement3 : spsThreePhaseVIMeasurementLib/Three-Phase V-I Measurement  VoltageMeasurement=phase-to-ground  SetLabelV=on  LabelV=Vabc  Vpu=on  VpuLL=off  CurrentMeasurement=yes  SetLabelI=on  LabelI=Iabc  Ipu=on  Pbase=100e6  Vbase=230e3  OutputType=Complex  PhasorSimulation=off  PSBequivalent=0
  Conn7 : PMIOPort  Side=Left
  Conn8 : PMIOPort  Port=2  Side=Left
  Conn9 : PMIOPort  Port=3  Side=Left
  Conn1 : PMIOPort  Port=4  Side=Right
  Conn2 : PMIOPort  Port=5  Side=Right
  Conn3 : PMIOPort  Port=6  Side=Right
  Conn4 : PMIOPort  Port=7  Side=Right
  Conn5 : PMIOPort  Port=8  Side=Right
  Conn6 : PMIOPort  Port=9  Side=Right
  Conn10 : PMIOPort  Port=10  Side=Left
  Conn11 : PMIOPort  Port=11  Side=Left
  Conn12 : PMIOPort  Port=12  Side=Left
  connections:
  Conn12/RConn1 -- Three-Phase V-I Measurement3/LConn3 -- Conn9/RConn1 -- Three-Phase V-I Measurement1/LConn3
  Conn11/RConn1 -- Three-Phase V-I Measurement3/LConn2 -- Conn8/RConn1 -- Three-Phase V-I Measurement1/LConn2
  Conn10/RConn1 -- Three-Phase V-I Measurement3/LConn1 -- Conn7/RConn1 -- Three-Phase V-I Measurement1/LConn1
  Three-Phase V-I Measurement3/RConn3 -- Conn6/RConn1
  Three-Phase V-I Measurement1/RConn3 -- Conn3/RConn1
  Three-Phase V-I Measurement1/RConn1 -- Conn1/RConn1
  Three-Phase V-I Measurement1/RConn2 -- Conn2/RConn1
  Three-Phase V-I Measurement3/RConn1 -- Conn4/RConn1
  Three-Phase V-I Measurement3/RConn2 -- Conn5/RConn1

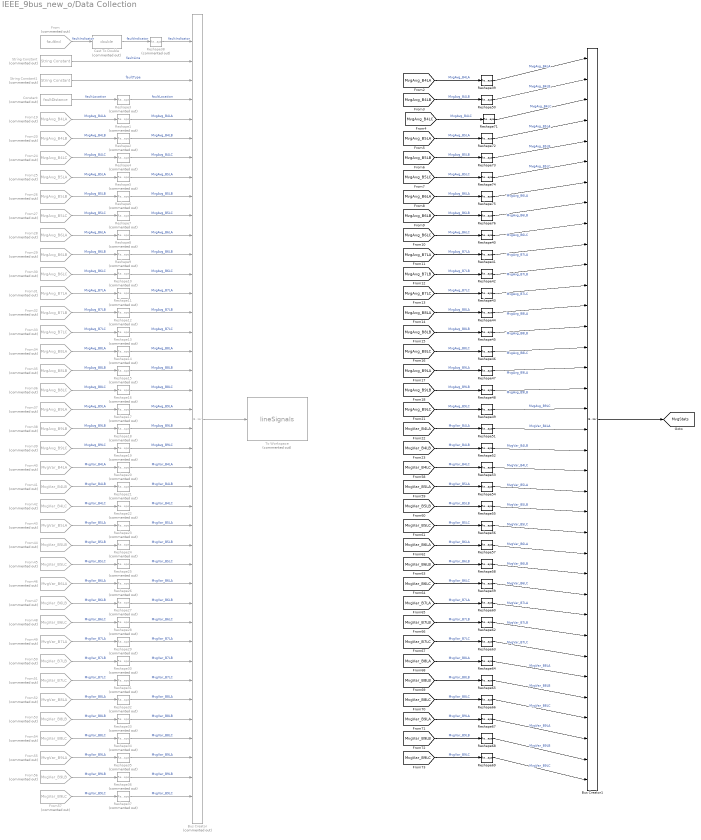
== system IEEE_9bus_new_o/Data Collection ==
  Bus Creator : BusCreator  Commented=on  Inputs=40
  Bus Creator1 : BusCreator  Inputs=36
  Cast To Double : DataTypeConversion  Commented=on  OutDataTypeStr=double  RndMeth=Round  SaturateOnIntegerOverflow=off
  Constant : Constant  Commented=on  Value=faultDistance
  From : From  Commented=on  GotoTag=faultInd  TagVisibility=global
  From19 : From  Commented=on  GotoTag=MvgAvg_B4LA  TagVisibility=global
  From20 : From  Commented=on  GotoTag=MvgAvg_B4LB  TagVisibility=global
  From24 : From  Commented=on  GotoTag=MvgAvg_B4LC  TagVisibility=global
  From25 : From  Commented=on  GotoTag=MvgAvg_B5LA  TagVisibility=global
  From26 : From  Commented=on  GotoTag=MvgAvg_B5LB  TagVisibility=global
  From27 : From  Commented=on  GotoTag=MvgAvg_B5LC  TagVisibility=global
  From28 : From  Commented=on  GotoTag=MvgAvg_B6LA  TagVisibility=global
  From29 : From  Commented=on  GotoTag=MvgAvg_B6LB  TagVisibility=global
  From30 : From  Commented=on  GotoTag=MvgAvg_B6LC  TagVisibility=global
  From31 : From  Commented=on  GotoTag=MvgAvg_B7LA  TagVisibility=global
  From32 : From  Commented=on  GotoTag=MvgAvg_B7LB  TagVisibility=global
  From33 : From  Commented=on  GotoTag=MvgAvg_B7LC  TagVisibility=global
  From34 : From  Commented=on  GotoTag=MvgAvg_B8LA  TagVisibility=global
  From35 : From  Commented=on  GotoTag=MvgAvg_B8LB  TagVisibility=global
  From36 : From  Commented=on  GotoTag=MvgAvg_B8LC  TagVisibility=global
  From37 : From  Commented=on  GotoTag=MvgAvg_B9LA  TagVisibility=global
  From38 : From  Commented=on  GotoTag=MvgAvg_B9LB  TagVisibility=global
  From39 : From  Commented=on  GotoTag=MvgAvg_B9LC  TagVisibility=global
  From40 : From  Commented=on  GotoTag=MvgVar_B4LA  TagVisibility=global
  From41 : From  Commented=on  GotoTag=MvgVar_B4LB  TagVisibility=global
  From42 : From  Commented=on  GotoTag=MvgVar_B4LC  TagVisibility=global
  From43 : From  Commented=on  GotoTag=MvgVar_B5LA  TagVisibility=global
  From44 : From  Commented=on  GotoTag=MvgVar_B5LB  TagVisibility=global
  From45 : From  Commented=on  GotoTag=MvgVar_B5LC  TagVisibility=global
  From46 : From  Commented=on  GotoTag=MvgVar_B6LA  TagVisibility=global
  From47 : From  Commented=on  GotoTag=MvgVar_B6LB  TagVisibility=global
  From48 : From  Commented=on  GotoTag=MvgVar_B6LC  TagVisibility=global
  From49 : From  Commented=on  GotoTag=MvgVar_B7LA  TagVisibility=global
  From50 : From  Commented=on  GotoTag=MvgVar_B7LB  TagVisibility=global
  From51 : From  Commented=on  GotoTag=MvgVar_B7LC  TagVisibility=global
  From52 : From  Commented=on  GotoTag=MvgVar_B8LA  TagVisibility=global
  From53 : From  Commented=on  GotoTag=MvgVar_B8LB  TagVisibility=global
  From54 : From  Commented=on  GotoTag=MvgVar_B8LC  TagVisibility=global
  From55 : From  Commented=on  GotoTag=MvgVar_B9LA  TagVisibility=global
  From56 : From  Commented=on  GotoTag=MvgVar_B9LB  TagVisibility=global
  From57 : From  Commented=on  GotoTag=MvgVar_B9LC  TagVisibility=global
  Reshape{1..38} (38 alike) : Reshape  Commented=on  OutputDimensionality=Customize  OutputDimensions=1
  Reshape{39..60,62..69,71..76} (36 alike) : Reshape  OutputDimensionality=Customize  OutputDimensions=1
  String Constant : StringConstant  Commented=on  String=faultLineStr
  String Constant1 : StringConstant  Commented=on  String=faultType
  To Workspace : ToWorkspace  Commented=on  VariableName=lineSignals  SaveFormat=Timeseries  SampleTime=-1
      settings: Save2DSignal=2-D array (concatenate along first dimension)
  tag scope: MvgStats=global
  wires:
  From35/1 -> Reshape15/1  "MvgAvg_B8LB"
  From19/1 -> Reshape1/1  "MvgAvg_B4LA"
  From43/1 -> Reshape23/1  "MvgVar_B5LA"
  From25/1 -> Reshape5/1  "MvgAvg_B5LA"
  From20/1 -> Reshape2/1  "MvgAvg_B4LB"
  From34/1 -> Reshape14/1  "MvgAvg_B8LA"
  From36/1 -> Reshape16/1  "MvgAvg_B8LC"
  From48/1 -> Reshape28/1  "MvgVar_B6LC"
  From42/1 -> Reshape22/1  "MvgVar_B4LC"
  Bus Creator/1 -> To Workspace/1
  From26/1 -> Reshape6/1  "MvgAvg_B5LB"
  From56/1 -> Reshape36/1  "MvgVar_B9LB"
  From57/1 -> Reshape37/1  "MvgVar_B9LC"
  From53/1 -> Reshape33/1  "MvgVar_B8LB"
  From37/1 -> Reshape17/1  "MvgAvg_B9LA"
  From46/1 -> Reshape26/1  "MvgVar_B6LA"
  From31/1 -> Reshape11/1  "MvgAvg_B7LA"
  From47/1 -> Reshape27/1  "MvgVar_B6LB"
  From29/1 -> Reshape9/1  "MvgAvg_B6LB"
  From33/1 -> Reshape13/1  "MvgAvg_B7LC"
  From49/1 -> Reshape29/1  "MvgVar_B7LA"
  From54/1 -> Reshape34/1  "MvgVar_B8LC"
  From38/1 -> Reshape18/1  "MvgAvg_B9LB"
  From55/1 -> Reshape35/1  "MvgVar_B9LA"
  String Constant/1 -> Bus Creator/2  "faultLine"
  From30/1 -> Reshape10/1  "MvgAvg_B6LC"
  From44/1 -> Reshape24/1  "MvgVar_B5LB"
  From39/1 -> Reshape19/1  "MvgAvg_B9LC"
  From41/1 -> Reshape21/1  "MvgVar_B4LB"
  From27/1 -> Reshape7/1  "MvgAvg_B5LC"
  From51/1 -> Reshape31/1  "MvgVar_B7LC"
  From45/1 -> Reshape25/1  "MvgVar_B5LC"
  From40/1 -> Reshape20/1  "MvgVar_B4LA"
  Constant/1 -> Reshape3/1  "faultLocation"
  From28/1 -> Reshape8/1  "MvgAvg_B6LA"
  From24/1 -> Reshape4/1  "MvgAvg_B4LC"
  From50/1 -> Reshape30/1  "MvgVar_B7LB"
  From52/1 -> Reshape32/1  "MvgVar_B8LA"
  From32/1 -> Reshape12/1  "MvgAvg_B7LB"
  String Constant1/1 -> Bus Creator/3  "faultType"
  Reshape3/1 -> Bus Creator/4  "faultLocation"
  Reshape1/1 -> Bus Creator/5  "MvgAvg_B4LA"
  Reshape2/1 -> Bus Creator/6  "MvgAvg_B4LB"
  Reshape4/1 -> Bus Creator/7  "MvgAvg_B4LC"
  Reshape5/1 -> Bus Creator/8  "MvgAvg_B5LA"
  Reshape6/1 -> Bus Creator/9  "MvgAvg_B5LB"
  Reshape7/1 -> Bus Creator/10  "MvgAvg_B5LC"
  Reshape8/1 -> Bus Creator/11  "MvgAvg_B6LA"
  Reshape9/1 -> Bus Creator/12  "MvgAvg_B6LB"
  Reshape10/1 -> Bus Creator/13  "MvgAvg_B6LC"
  Reshape11/1 -> Bus Creator/14  "MvgAvg_B7LA"
  Reshape12/1 -> Bus Creator/15  "MvgAvg_B7LB"
  Reshape13/1 -> Bus Creator/16  "MvgAvg_B7LC"
  Reshape14/1 -> Bus Creator/17  "MvgAvg_B8LA"
  Reshape15/1 -> Bus Creator/18  "MvgAvg_B8LB"
  Reshape16/1 -> Bus Creator/19  "MvgAvg_B8LC"
  Reshape17/1 -> Bus Creator/20  "MvgAvg_B9LA"
  Reshape18/1 -> Bus Creator/21  "MvgAvg_B9LB"
  Reshape19/1 -> Bus Creator/22  "MvgAvg_B9LC"
  Reshape20/1 -> Bus Creator/23  "MvgVar_B4LA"
  Reshape21/1 -> Bus Creator/24  "MvgVar_B4LB"
  Reshape22/1 -> Bus Creator/25  "MvgVar_B4LC"
  Reshape23/1 -> Bus Creator/26  "MvgVar_B5LA"
  Reshape24/1 -> Bus Creator/27  "MvgVar_B5LB"
  Reshape25/1 -> Bus Creator/28  "MvgVar_B5LC"
  Reshape26/1 -> Bus Creator/29  "MvgVar_B6LA"
  Reshape27/1 -> Bus Creator/30  "MvgVar_B6LB"
  Reshape28/1 -> Bus Creator/31  "MvgVar_B6LC"
  Reshape29/1 -> Bus Creator/32  "MvgVar_B7LA"
  Reshape30/1 -> Bus Creator/33  "MvgVar_B7LB"
  Reshape31/1 -> Bus Creator/34  "MvgVar_B7LC"
  Reshape32/1 -> Bus Creator/35  "MvgVar_B8LA"
  Reshape33/1 -> Bus Creator/36  "MvgVar_B8LB"
  Reshape34/1 -> Bus Creator/37  "MvgVar_B8LC"
  Reshape35/1 -> Bus Creator/38  "MvgVar_B9LA"
  Reshape36/1 -> Bus Creator/39  "MvgVar_B9LB"
  Reshape37/1 -> Bus Creator/40  "MvgVar_B9LC"
  From/1 -> Cast To Double/1  "faultIndicator"
  Cast To Double/1 -> Reshape38/1  "faultIndicator"
  Reshape38/1 -> Bus Creator/1  "faultIndicator"
  Reshape69/1 -> Bus Creator1/36  "MvgVar_B9LC"
  Reshape68/1 -> Bus Creator1/35  "MvgVar_B9LB"
  Reshape67/1 -> Bus Creator1/34  "MvgVar_B9LA"
  Reshape66/1 -> Bus Creator1/33  "MvgVar_B8LC"
  Reshape65/1 -> Bus Creator1/32  "MvgVar_B8LB"
  Reshape64/1 -> Bus Creator1/31  "MvgVar_B8LA"
  Reshape63/1 -> Bus Creator1/30  "MvgVar_B7LC"
  Reshape62/1 -> Bus Creator1/29  "MvgVar_B7LB"
  Reshape60/1 -> Bus Creator1/28  "MvgVar_B7LA"
  Reshape59/1 -> Bus Creator1/27  "MvgVar_B6LC"
  Reshape58/1 -> Bus Creator1/26  "MvgVar_B6LB"
  Reshape57/1 -> Bus Creator1/25  "MvgVar_B6LA"
  Reshape56/1 -> Bus Creator1/24  "MvgVar_B5LC"
  Reshape55/1 -> Bus Creator1/23  "MvgVar_B5LB"
  Reshape54/1 -> Bus Creator1/22  "MvgVar_B5LA"
  Reshape53/1 -> Bus Creator1/21  "MvgVar_B4LC"
  Reshape52/1 -> Bus Creator1/20  "MvgVar_B4LB"
  Reshape51/1 -> Bus Creator1/19  "MvgVar_B4LA"
  Reshape49/1 -> Bus Creator1/18  "MvgAvg_B9LC"
  Reshape48/1 -> Bus Creator1/17  "MvgAvg_B9LB"
  Reshape47/1 -> Bus Creator1/16  "MvgAvg_B9LA"
  Reshape46/1 -> Bus Creator1/15  "MvgAvg_B8LC"
  Reshape45/1 -> Bus Creator1/14  "MvgAvg_B8LB"
  Reshape44/1 -> Bus Creator1/13  "MvgAvg_B8LA"
  Reshape43/1 -> Bus Creator1/12  "MvgAvg_B7LC"
  Reshape42/1 -> Bus Creator1/11  "MvgAvg_B7LB"
  Reshape41/1 -> Bus Creator1/10  "MvgAvg_B7LA"
  Reshape40/1 -> Bus Creator1/9  "MvgAvg_B6LC"
  Reshape76/1 -> Bus Creator1/8  "MvgAvg_B6LB"
  Reshape75/1 -> Bus Creator1/7  "MvgAvg_B6LA"
  Reshape74/1 -> Bus Creator1/6  "MvgAvg_B5LC"
  Reshape73/1 -> Bus Creator1/5  "MvgAvg_B5LB"
  Reshape72/1 -> Bus Creator1/4  "MvgAvg_B5LA"
  Reshape71/1 -> Bus Creator1/3  "MvgAvg_B4LC"
  Reshape50/1 -> Bus Creator1/2  "MvgAvg_B4LB"
  Reshape39/1 -> Bus Creator1/1  "MvgAvg_B4LA"
  [MvgAvg_B7LB] -> Reshape42/1  "MvgAvg_B7LB"
  [MvgVar_B8LA] -> Reshape64/1  "MvgVar_B8LA"
  [MvgVar_B7LB] -> Reshape62/1  "MvgVar_B7LB"
  [MvgAvg_B4LC] -> Reshape71/1  "MvgAvg_B4LC"
  [MvgAvg_B6LA] -> Reshape75/1  "MvgAvg_B6LA"
  [MvgVar_B4LA] -> Reshape51/1  "MvgVar_B4LA"
  [MvgVar_B5LC] -> Reshape56/1  "MvgVar_B5LC"
  [MvgVar_B7LC] -> Reshape63/1  "MvgVar_B7LC"
  [MvgAvg_B5LC] -> Reshape74/1  "MvgAvg_B5LC"
  [MvgVar_B4LB] -> Reshape52/1  "MvgVar_B4LB"
  [MvgAvg_B9LC] -> Reshape49/1  "MvgAvg_B9LC"
  [MvgVar_B5LB] -> Reshape55/1  "MvgVar_B5LB"
  [MvgAvg_B6LC] -> Reshape40/1  "MvgAvg_B6LC"
  [MvgVar_B9LA] -> Reshape67/1  "MvgVar_B9LA"
  [MvgAvg_B9LB] -> Reshape48/1  "MvgAvg_B9LB"
  [MvgVar_B8LC] -> Reshape66/1  "MvgVar_B8LC"
  [MvgVar_B7LA] -> Reshape60/1  "MvgVar_B7LA"
  [MvgAvg_B7LC] -> Reshape43/1  "MvgAvg_B7LC"
  [MvgAvg_B6LB] -> Reshape76/1  "MvgAvg_B6LB"
  [MvgVar_B6LB] -> Reshape58/1  "MvgVar_B6LB"
  [MvgAvg_B7LA] -> Reshape41/1  "MvgAvg_B7LA"
  [MvgVar_B6LA] -> Reshape57/1  "MvgVar_B6LA"
  [MvgAvg_B9LA] -> Reshape47/1  "MvgAvg_B9LA"
  [MvgVar_B8LB] -> Reshape65/1  "MvgVar_B8LB"
  [MvgVar_B9LC] -> Reshape69/1  "MvgVar_B9LC"
  [MvgVar_B9LB] -> Reshape68/1  "MvgVar_B9LB"
  [MvgAvg_B5LB] -> Reshape73/1  "MvgAvg_B5LB"
  Bus Creator1/1 -> [MvgStats]
  [MvgVar_B4LC] -> Reshape53/1  "MvgVar_B4LC"
  [MvgVar_B6LC] -> Reshape59/1  "MvgVar_B6LC"
  [MvgAvg_B8LC] -> Reshape46/1  "MvgAvg_B8LC"
  [MvgAvg_B8LA] -> Reshape44/1  "MvgAvg_B8LA"
  [MvgAvg_B4LB] -> Reshape50/1  "MvgAvg_B4LB"
  [MvgAvg_B5LA] -> Reshape72/1  "MvgAvg_B5LA"
  [MvgVar_B5LA] -> Reshape54/1  "MvgVar_B5LA"
  [MvgAvg_B4LA] -> Reshape39/1  "MvgAvg_B4LA"
  [MvgAvg_B8LB] -> Reshape45/1  "MvgAvg_B8LB"
